simulink model "monofasikos_ask5_2kai3_monofasikos"  (R2021a)
settings: Solver=ode23tb  StartTime=0.0  StopTime=7.2  MaxStep=1e-5  RelTol=1e-3
libraries: spsRMSLib x7, spsCurrentMeasurementLib x4, spsSaturableTransformerLib x3, spsVoltageMeasurementLib x3, spsControlledVoltageSourceLib x2, simulink x2, spsPowerLib x2, spsSeriesRLCBranchLib x1, spsDCVoltageSourceLib x1, spspowerguiLib x1
settings Model: Creator=User  LastModifiedBy=alexi
settings SolverCC: AlgebraicLoopSolver=TrustRegion
settings DebuggingCC: SFMachineParentedDataDiag=warning

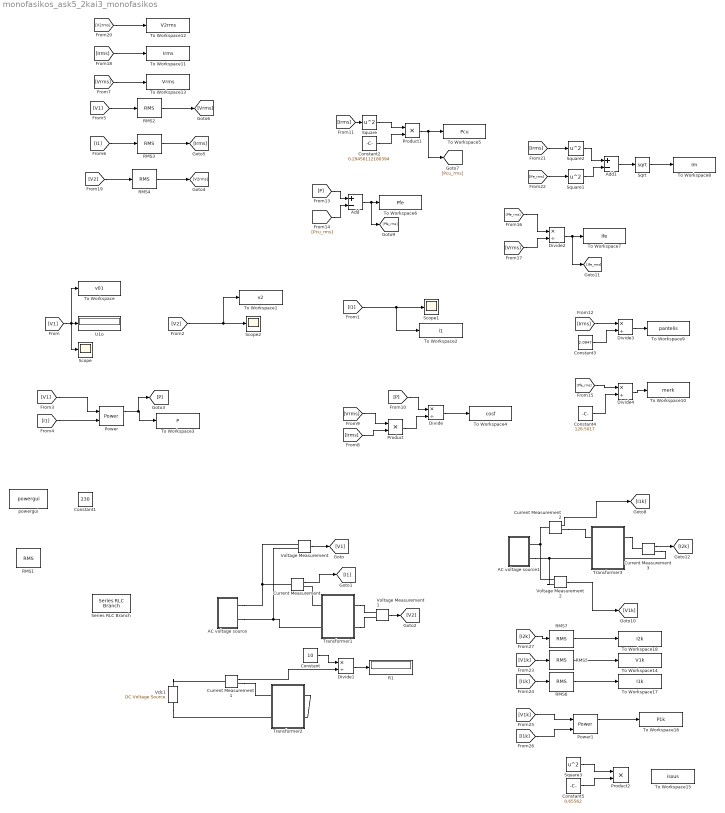
== system monofasikos_ask5_2kai3_monofasikos ==
  AC voltage source : Subsystem  mask{Vrms=230}
  AC voltage source1 : Subsystem  mask{Vrms=200}
  Add : Sum  Inputs=+-
  Add1 : Sum  Inputs=+-
  Constant : Constant  Value=10
  Constant1 : Constant  Value=230
  Constant2 : Constant  Value=0.29456112180394
  Constant3 : Constant  Value=2.0947
  Constant4 : Constant  Value=126.5017
  Constant5 : Constant  Value=0.65562
  Current Measurement{,1..3} (4 alike) : spsCurrentMeasurementLib/Current Measurement  PhasorSimulation=off  OutputType=Complex  PSBequivalent=0
  Divide{,1..4} (5 alike) : Product  Inputs=*/
  Power : spsPowerLib/Power  Freq=50  Vinit=[0, 0]  Iinit=[0, 0]  Ts=1e-5
      settings: SourceProductBaseCode=PS
  Power1 : spsPowerLib/Power  Freq=50  Vinit=[0, 0]  Iinit=[0, 0]  Ts=1e-5
      settings: SourceProductBaseCode=PS
  Product : Product
  Product1 : Product
  Product2 : Product
  R1 : Display
  RMS{1..7} (7 alike) : spsRMSLib/RMS  TrueRMS=on  Freq=50  RMSInit=0  Ts=0
  Scope : Scope
  Scope1 : Scope
  Scope2 : Scope
  Series RLC Branch : spsSeriesRLCBranchLib/Series RLC Branch  LConnTagsString=__new0  RConnTagsString=__new0  BranchType=RLC  Resistance=1  Inductance=1e-3  SetiL0=off  InitialCurrent=0  Capacitance=1e-6  Setx0=off  InitialVoltage=0  Measurements=None
  Sqrt : Sqrt  SaturateOnIntegerOverflow=on
  Square{,1..3} (4 alike) : Math  Operator=square  SaturateOnIntegerOverflow=on
  To Workspace : ToWorkspace  VariableName=v01  SaveFormat=Timeseries  SampleTime=1e-5
  To Workspace1 : ToWorkspace  VariableName=v2  SaveFormat=Timeseries  SampleTime=1e-5
  To Workspace10 : ToWorkspace  VariableName=merk  SaveFormat=Timeseries  SampleTime=1e-5
  To Workspace11 : ToWorkspace  VariableName=Irms  SaveFormat=Timeseries  SampleTime=1e-5
  To Workspace12 : ToWorkspace  VariableName=V2rms  SaveFormat=Timeseries  SampleTime=1e-5
  To Workspace13 : ToWorkspace  VariableName=Vrms  SaveFormat=Timeseries  SampleTime=1e-5
  To Workspace14 : ToWorkspace  VariableName=V1k  SaveFormat=Timeseries  SampleTime=1e-5
  To Workspace15 : ToWorkspace  VariableName=isxus  SaveFormat=Timeseries  SampleTime=1e-5
  To Workspace16 : ToWorkspace  VariableName=P1k  SaveFormat=Timeseries  SampleTime=1e-5
  To Workspace17 : ToWorkspace  VariableName=I1k  SaveFormat=Timeseries  SampleTime=1e-5
  To Workspace18 : ToWorkspace  VariableName=I2k  SaveFormat=Timeseries  SampleTime=1e-5
  To Workspace2 : ToWorkspace  VariableName=i1  SaveFormat=Timeseries  SampleTime=1e-5
  To Workspace3 : ToWorkspace  VariableName=P  SaveFormat=Timeseries  SampleTime=1e-5
  To Workspace4 : ToWorkspace  VariableName=cosf  SaveFormat=Timeseries  SampleTime=1e-5
  To Workspace5 : ToWorkspace  VariableName=Pcu  SaveFormat=Timeseries  SampleTime=1e-5
  To Workspace6 : ToWorkspace  VariableName=Pfe  SaveFormat=Timeseries  SampleTime=1e-5
  To Workspace7 : ToWorkspace  VariableName=Ife  SaveFormat=Timeseries  SampleTime=1e-5
  To Workspace8 : ToWorkspace  VariableName=Im  SaveFormat=Timeseries  SampleTime=1e-5
  To Workspace9 : ToWorkspace  VariableName=pantelis  SaveFormat=Timeseries  SampleTime=1e-5
  Transformer1 : Subsystem  mask{PN=4, U1N=230, U2N=115}
      mask prompts: PN "PN (kVA)"; U1N "U1N (V)"; U2N "U2N (V)"
  Transformer2 : Subsystem  mask{PN=4, U1N=230, U2N=115}
      mask prompts: PN "PN (kVA)"; U1N "U1N (V)"; U2N "U2N (V)"
  Transformer3 : Subsystem  mask{PN=4, U1N=230, U2N=115}
      mask prompts: PN "PN (kVA)"; U1N "U1N (V)"; U2N "U2N (V)"
  U1o : Display
  Vdc1 : spsDCVoltageSourceLib/DC Voltage Source  Amplitude=10  Measurements=Voltage
  Voltage Measurement : spsVoltageMeasurementLib/Voltage Measurement  PhasorSimulation=off  OutputType=Complex  PSBequivalent=0
  Voltage Measurement1 : spsVoltageMeasurementLib/Voltage Measurement  PhasorSimulation=off  OutputType=Complex  PSBequivalent=0
  Voltage Measurement2 : spsVoltageMeasurementLib/Voltage Measurement  PhasorSimulation=off  OutputType=Complex  PSBequivalent=0
  powergui : spspowerguiLib/powergui  Priority=1  SimulationMode=Continuous  SampleTime=50e-6  frequency=60  Iterations=50  frequencyindice=0  Pbase=100e6  ErrMax=1e-4  UnitsV=kV  UnitsW=MW  buscounter=0  FunctionMessages=off  echomessages=off  EnableUseOfTLC=off  CurrentSourceSwitches=off  DisableSnubberDevices=off  DisableRonSwitches=off  DisableVfSwitches=off  DisplayEquations=off  AutomaticDiscreteSolvers=off  SolverType=Tustin/Backward Euler (TBE)  Interpol=off  ExternalGateDelay=off  methode=off  Ts=100  x0status=blocks  SPID=on  SwTol=0  HookPort=off  NonlinearTolerance=1e-4  nMaxIteration=100  ContinueOnMaxIteration=off  RestoreLinks=warning  ResistiveCurrentMeasurement=off  Frange=[0:2:500]  Ylog=off  Xlog=on  ShowGrid=off  save=off  variable=ZData  structure=0  ZoomFFT=off  StartTime=0.0  cycles=1  DisplayStyle=1  fundamental=60  FreqAxis=off  MaxFrequency=1000  frequencyindicesteady=1  RmsSteady=1  display=off
  wires:
  Voltage Measurement/1 -> [V1]
  Current Measurement/1 -> [I1]
  Voltage Measurement1/1 -> [V2]
  [V1] -> Scope/1, To Workspace/1, U1o/1
  [I1] -> To Workspace2/1, Scope1/1
  [V2] -> To Workspace1/1, Scope2/1
  [V1] -> Power/1
  [I1] -> Power/2
  Power/1 -> [P], To Workspace3/1
  [V1] -> RMS2/1
  [I1] -> RMS3/1
  RMS2/1 -> [Vrms]
  RMS3/1 -> [Irms]
  [Vrms] -> Product/1
  [Irms] -> Product/2
  Product/1 -> Divide/2
  [P] -> Divide/1
  Divide/1 -> To Workspace4/1
  [Irms] -> Square/1
  Current Measurement1/1 -> Divide1/2
  Constant/1 -> Divide1/1
  Divide1/1 -> R1/1
  Square/1 -> Product1/1
  Constant2/1 -> Product1/2
  Product1/1 -> [Pcu_rms], To Workspace5/1
  [P] -> Add/1
  [Pcu_rms] -> Add/2
  Add/1 -> [Pfe_rms], To Workspace6/1
  [Pfe_rms] -> Divide2/1
  [Vrms] -> Divide2/2
  Divide2/1 -> [Ife_rms], To Workspace7/1
  [Irms] -> Square2/1
  [Ife_rms] -> Square1/1
  Square2/1 -> Add1/1
  Square1/1 -> Add1/2
  Add1/1 -> Sqrt/1
  Sqrt/1 -> To Workspace8/1
  [Irms] -> Divide3/1
  Constant3/1 -> Divide3/2
  Divide3/1 -> To Workspace9/1
  [Pfe_rms] -> Divide4/1
  Divide4/1 -> To Workspace10/1
  Constant4/1 -> Divide4/2
  [Irms] -> To Workspace11/1
  [Vrms] -> To Workspace13/1
  RMS4/1 -> [V2rms]
  [V2] -> RMS4/1
  [V2rms] -> To Workspace12/1
  Voltage Measurement2/1 -> [V1k]
  Square3/1 -> Product2/1
  Constant5/1 -> Product2/2
  [V1k] -> Power1/1
  [I1k] -> Power1/2
  Power1/1 -> To Workspace16/1
  Current Measurement2/1 -> [I1k]
  [V1k] -> RMS5/1
  RMS5/1 -> To Workspace14/1
  [I1k] -> RMS6/1
  RMS6/1 -> To Workspace17/1
  [I2k] -> RMS7/1
  RMS7/1 -> To Workspace18/1
  Current Measurement3/1 -> [I2k]
  connections:
  AC voltage source/RConn1 -- Current Measurement/LConn1 -- Voltage Measurement/LConn1
  AC voltage source/RConn2 -- Voltage Measurement/LConn2 -- Transformer1/LConn2
  Transformer1/RConn1 -- Voltage Measurement1/LConn1
  Transformer1/RConn2 -- Voltage Measurement1/LConn2
  Vdc1/LConn1 -- Transformer2/LConn2
  Transformer1/LConn1 -- Current Measurement/RConn1
  Vdc1/RConn1 -- Current Measurement1/LConn1
  Current Measurement1/RConn1 -- Transformer2/LConn1
  Transformer2/RConn1 -- Transformer2/RConn2
  AC voltage source1/RConn2 -- Voltage Measurement2/LConn2 -- Transformer3/LConn2
  Voltage Measurement2/LConn1 -- Current Measurement2/LConn1 -- AC voltage source1/RConn1
  Current Measurement2/RConn1 -- Transformer3/LConn1
  Transformer3/RConn1 -- Current Measurement3/LConn1
  Current Measurement3/RConn1 -- Transformer3/RConn2

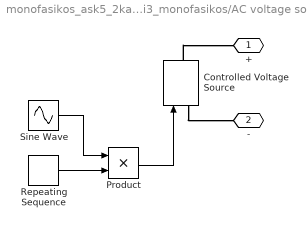
== system monofasikos_ask5_2kai3_monofasikos/AC voltage source ==
  Controlled Voltage Source : spsControlledVoltageSourceLib/Controlled Voltage Source  Initialize=on  Source_Type=AC  Amplitude=0  Phase=0  Frequency=50  Measurements=Voltage
  Product : Product
  Repeating Sequence : simulink/Sources/Repeating Sequence  rep_seq_t=t  rep_seq_y=Vs
  Sine Wave : Sin  Amplitude=sqrt(2)  Frequency=100*pi  SampleTime=0
  + : PMIOPort  Side=Right
  - : PMIOPort  Port=2  Side=Right
  wires:
  Product/1 -> Controlled Voltage Source/1
  Sine Wave/1 -> Product/1
  Repeating Sequence/1 -> Product/2
  connections:
  Controlled Voltage Source/LConn1 -- -/RConn1
  Controlled Voltage Source/RConn1 -- +/RConn1

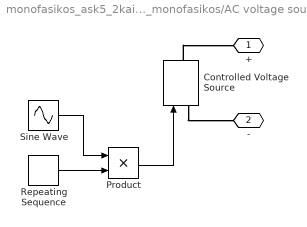
== system monofasikos_ask5_2kai3_monofasikos/AC voltage source1 ==
  Controlled Voltage Source : spsControlledVoltageSourceLib/Controlled Voltage Source  Initialize=on  Source_Type=AC  Amplitude=0  Phase=0  Frequency=50  Measurements=Voltage
  Product : Product
  Repeating Sequence : simulink/Sources/Repeating Sequence  rep_seq_t=t  rep_seq_y=Vs
  Sine Wave : Sin  Amplitude=sqrt(2)  Frequency=100*pi  SampleTime=0
  + : PMIOPort  Side=Right
  - : PMIOPort  Port=2  Side=Right
  wires:
  Product/1 -> Controlled Voltage Source/1
  Sine Wave/1 -> Product/1
  Repeating Sequence/1 -> Product/2
  connections:
  Controlled Voltage Source/LConn1 -- -/RConn1
  Controlled Voltage Source/RConn1 -- +/RConn1

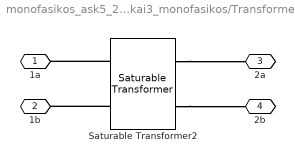
== system monofasikos_ask5_2kai3_monofasikos/Transformer1 ==
  Saturable Transformer2 : spsSaturableTransformerLib/Saturable Transformer  ThreeWindings=off  Hysteresis=off  DataFile='hysteresis.mat'  Measurements=None  UNITS=pu  NominalPower=[4e3 50]  Winding1=[230 0.022273 0.015903]  Winding2=[122 0.024298 0.019083]  Winding3=[3.15e+05 0.00245 0.098001]  Saturation=[0 0;0.031714 0.76205;0.037813 0.86926;0.045538 0.94653;0.060175 1.0141;0.080911 1.0624;0.14637 1.159]  CoreLoss=35.539  BreakLoop=off  DiscreteSolver=Trapezoidal iterative  DataType=off  InitialFlux=0  TransfoNumber=1
      settings: SourceProductBaseCode=PS
  1a : PMIOPort  Side=Left
  1b : PMIOPort  Port=2  Side=Left
  2a : PMIOPort  Port=3  Side=Right
  2b : PMIOPort  Port=4  Side=Right
  connections:
  Saturable Transformer2/RConn2 -- 2b/RConn1
  Saturable Transformer2/LConn1 -- 1a/RConn1
  Saturable Transformer2/RConn1 -- 2a/RConn1
  Saturable Transformer2/LConn2 -- 1b/RConn1

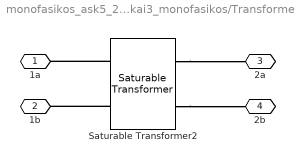
== system monofasikos_ask5_2kai3_monofasikos/Transformer2 ==
  Saturable Transformer2 : spsSaturableTransformerLib/Saturable Transformer  ThreeWindings=off  Hysteresis=off  DataFile='hysteresis.mat'  Measurements=None  UNITS=SI  NominalPower=[4e3 50]  Winding1=[230 0.29456 0.00066946]  Winding2=[122 0.090413 0.00022602]  Winding3=[3.15e+05 60775 7738.2]  Saturation=[0 0;0.78001 0.789;0.93001 0.9;1.12 0.98;1.48 1.05;1.99 1.1;3.6 1.2]  CoreLoss=470  BreakLoop=off  DiscreteSolver=Trapezoidal iterative  DataType=on  InitialFlux=0  TransfoNumber=1
      settings: SourceProductBaseCode=PS
  1a : PMIOPort  Side=Left
  1b : PMIOPort  Port=2  Side=Left
  2a : PMIOPort  Port=3  Side=Right
  2b : PMIOPort  Port=4  Side=Right
  connections:
  Saturable Transformer2/RConn2 -- 2b/RConn1
  Saturable Transformer2/LConn1 -- 1a/RConn1
  Saturable Transformer2/RConn1 -- 2a/RConn1
  Saturable Transformer2/LConn2 -- 1b/RConn1

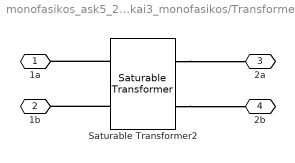
== system monofasikos_ask5_2kai3_monofasikos/Transformer3 ==
  Saturable Transformer2 : spsSaturableTransformerLib/Saturable Transformer  ThreeWindings=off  Hysteresis=off  DataFile='hysteresis.mat'  Measurements=None  UNITS=SI  NominalPower=[4e3 50]  Winding1=[230 0.29456 0.00066946]  Winding2=[122 0.090413 0.00022602]  Winding3=[3.15e+05 60775 7738.2]  Saturation=[0 0;0.78001 0.789;0.93001 0.9;1.12 0.98;1.48 1.05;1.99 1.1;3.6 1.2]  CoreLoss=470  BreakLoop=off  DiscreteSolver=Trapezoidal iterative  DataType=on  InitialFlux=0  TransfoNumber=1
      settings: SourceProductBaseCode=PS
  1a : PMIOPort  Side=Left
  1b : PMIOPort  Port=2  Side=Left
  2a : PMIOPort  Port=3  Side=Right
  2b : PMIOPort  Port=4  Side=Right
  connections:
  Saturable Transformer2/RConn2 -- 2b/RConn1
  Saturable Transformer2/LConn1 -- 1a/RConn1
  Saturable Transformer2/RConn1 -- 2a/RConn1
  Saturable Transformer2/LConn2 -- 1b/RConn1
